simulink model "model1"  (R2018b)
settings: Solver=VariableStepAuto  StartTime=0.0  StopTime=10.0  RelTol=1e-3
values from neighbouring files (symbols this model uses):
  A = [0 0 1 0; 0 0 0 1 ... (first row only)    [main1.m]
  B = [0;0;0;1/m2]    [main1.m]
  C = [0, 1, 0, 0]    [main1.m]
  K = place( A,B, p1)    [main1.m]
  L = place( A', C', p2)'    [main1.m]
settings Model: Creator=tim  LastModifiedBy=tim

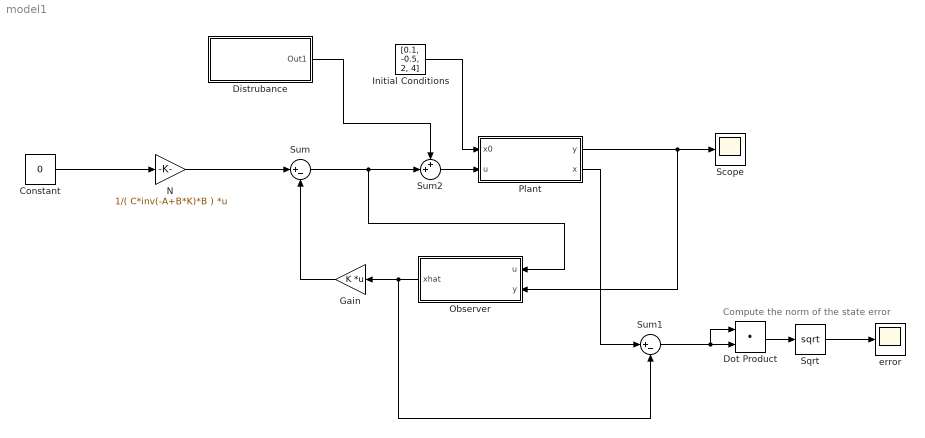
== system model1 ==
  note: Compute the norm of the state error
  Constant : Constant  Value=0
  Distrubance : Subsystem
  Dot Product : DotProduct  InputSameDT=on  OutDataTypeStr=Inherit: Inherit via internal rule
  Gain : Gain  Gain=K  Multiplication=Matrix(K*u)
  Initial Conditions : Constant  Value=[0.1, -0.5, 2, 4]
  N : Gain  Gain=1/( C*inv(-A+B*K)*B )  Multiplication=Matrix(K*u)
  "Observer " : Subsystem
  Plant : Subsystem
  Scope : Scope
  Sqrt : Sqrt  SaturateOnIntegerOverflow=on
  Sum : Sum  Inputs=|+-
  Sum1 : Sum  Inputs=|+-
  Sum2 : Sum  Inputs=++|
  error : Scope
  wires:
  Plant/1("y ") -> Scope/1, "Observer "/2(y)
  Initial Conditions/1 -> Plant/1(x0)
  "Observer "/1(xhat) -> Gain/1, Sum1/2
  Constant/1 -> N/1
  Sum/1 -> Sum2/2, "Observer "/1(u)
  Gain/1 -> Sum/2
  Plant/2(x) -> Sum1/1
  Sum1/1 -> Dot Product/1, Dot Product/2
  Dot Product/1 -> Sqrt/1
  Sqrt/1 -> error/1
  N/1 -> Sum/1
  Sum2/1 -> Plant/2(u)
  Distrubance/1(Out1) -> Sum2/1

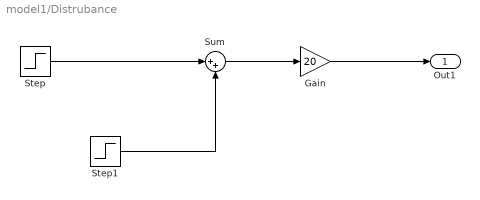
== system model1/Distrubance ==
  Gain : Gain  Gain=20
  Step : Step  Time=5  SampleTime=0
  Step1 : Step  Time=5.1  After=-1  SampleTime=0
  Sum : Sum  Inputs=|++
  Out1 : Outport
  wires:
  Step/1 -> Sum/1
  Step1/1 -> Sum/2
  Sum/1 -> Gain/1
  Gain/1 -> Out1/1

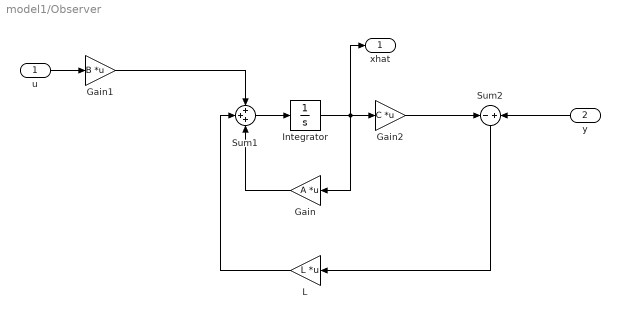
== system model1/Observer  ==
  u : Inport
  y : Inport  Port=2
  Gain : Gain  Gain=A  Multiplication=Matrix(K*u)
  Gain1 : Gain  Gain=B  Multiplication=Matrix(K*u)
  Gain2 : Gain  Gain=C  Multiplication=Matrix(K*u)
  Integrator : Integrator
  L : Gain  Gain=L  Multiplication=Matrix(K*u)
  Sum1 : Sum  Inputs=+++
  Sum2 : Sum  Inputs=-|+
  xhat : Outport
  wires:
  Integrator/1 -> xhat/1, Gain2/1, Gain/1
  Gain1/1 -> Sum1/1
  u/1 -> Gain1/1
  Gain2/1 -> Sum2/1
  Sum1/1 -> Integrator/1
  Gain/1 -> Sum1/3
  L/1 -> Sum1/2
  y/1 -> Sum2/2
  Sum2/1 -> L/1

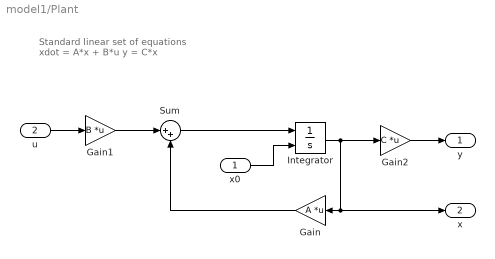
== system model1/Plant ==
  note: Standard linear set of equations
      | xdot = A*x + B*u
      | y = C*x
  x0 : Inport
  u : Inport  Port=2
  Gain : Gain  Gain=A  Multiplication=Matrix(K*u)
  Gain1 : Gain  Gain=B  Multiplication=Matrix(K*u)
  Gain2 : Gain  Gain=C  Multiplication=Matrix(K*u)
  Integrator : Integrator  InitialConditionSource=external
  Sum : Sum  Inputs=|++
  "y " : Outport
  x : Outport  Port=2
  wires:
  Integrator/1 -> x/1, Gain/1, Gain2/1
  Gain2/1 -> "y "/1
  Sum/1 -> Integrator/1
  Gain/1 -> Sum/2
  Gain1/1 -> Sum/1
  x0/1 -> Integrator/2
  u/1 -> Gain1/1
